simulink model "atomicVsVirtual"  (R2013a)
settings: Solver=VariableStepDiscrete  StartTime=0.0  StopTime=10.0  RelTol=1e-3
settings Model: Creator=bbhattac  LastModifiedBy=bbhattac

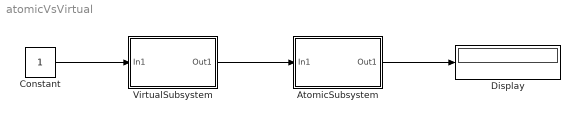
== system atomicVsVirtual ==
  AtomicSubsystem : Subsystem  TreatAsAtomicUnit=on
  Constant : Constant  SampleTime=0.1
  Display : Display
  VirtualSubsystem : Subsystem
  wires:
  Constant/1 -> VirtualSubsystem/1(In1)
  VirtualSubsystem/1(Out1) -> AtomicSubsystem/1(In1)
  AtomicSubsystem/1(Out1) -> Display/1

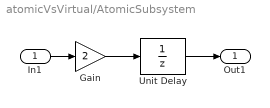
== system atomicVsVirtual/AtomicSubsystem ==
  In1 : Inport
  Gain : Gain  Gain=2
  Unit Delay : UnitDelay  SampleTime=-1
  Out1 : Outport
  wires:
  Gain/1 -> Unit Delay/1
  In1/1 -> Gain/1
  Unit Delay/1 -> Out1/1

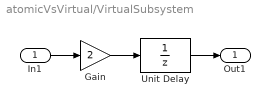
== system atomicVsVirtual/VirtualSubsystem ==
  In1 : Inport
  Gain : Gain  Gain=2
  Unit Delay : UnitDelay  SampleTime=-1
  Out1 : Outport
  wires:
  Unit Delay/1 -> Out1/1
  In1/1 -> Gain/1
  Gain/1 -> Unit Delay/1
